simulink model "carsim_seed_model"  (R2024b)
settings: Solver=ode45  StartTime=0  StopTime=12  FixedStep=0.002  RelTol=1e-3  AbsTol=1e-6
libraries: Solver_SF x1
settings Model: Creator=ywata  LastModifiedBy=MrZang
settings SolverCC: AutoScaleAbsTol=off  AlgebraicLoopSolver=TrustRegion
settings DataIOCC: SaveFormat=Array  SignalLoggingSaveFormat=ModelDataLogs  ReturnWorkspaceOutputs=off  SignalLoggingName=sigsOut
settings OptimizationCC: BlockReduction=off  BooleanDataType=off  ExpressionDepthLimit=2147483647  LifeSpan=inf
settings DebuggingCC: SaveWithParameterizedLinksMsg=none  UnderspecifiedInitializationDetection=Classic  MergeDetectMultiDrivingBlocksExec=none  SignalResolutionControl=TryResolveAllWithWarning  MultiTaskDSMMsg=warning  MultiTaskCondExecSysMsg=none  FcnCallInpInsideContextMsg=warning  UnconnectedInputMsg=warning  UnconnectedOutputMsg=warning  UnconnectedLineMsg=warning  StateNameClashWarn=warning  SFUnexpectedBacktrackingDiag=warning  SFNoUnconditionalDefaultTransitionDiag=warning  SFExecutionAtInitializationDiag=none  ArithmeticOperatorsInVariantConditions=warning
settings HardwareCC: ProdBitPerPointer=32  ProdBitPerSizeT=32  ProdBitPerPtrDiffT=32  ProdLargestAtomicFloat=None  ProdIntDivRoundTo=Undefined  ProdEndianess=Unspecified  ProdWordSize=32  ProdHWDeviceType=32-bit Generic  TargetUnknown=on
settings ModelReferenceCC: PropagateSignalLabelsOutOfModel=off
settings SFSimCC: SimUseLocalCustomCode=off  CustomCodeUndefinedFunction=UseInterfaceOnly
settings RTWCC: TemplateMakefile=grt_vc.tmf  RTWUseLocalCustomCode=off  GPUComputeCapability=3.5
settings CodeAppCC: StateflowObjectComments=on
settings GRTTargetCC: TargetFcnLib=ansi_tfl_tmw.mat  TargetLangStandard=C89/C90 (ANSI)  CombineOutputUpdateFcns=off  GRTInterface=on
settings ConfigComp: CovMetricSettings=dw  CovSaveCumulativeToWorkspaceVar=on  CovSaveSingleToWorkspaceVar=on  CovExternalEMLEnable=off

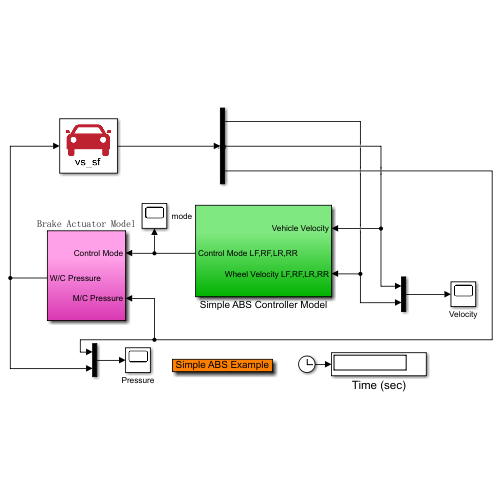
[thumbnail: Simulink's stored preview of the top-level diagram]
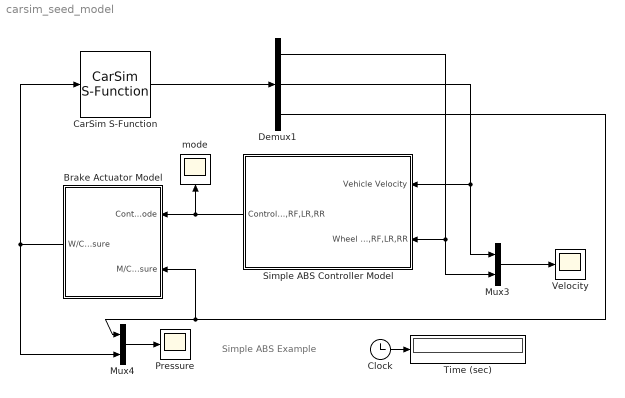
== system carsim_seed_model ==
  note: Simple ABS Example
  Brake Actuator Model : Subsystem
  CarSim S-Function : Solver_SF/CarSim S-Function  Priority=1  SIMFILE=simfile.sim
  Clock : Clock
  Demux1 : Demux  Outputs=[4 1 1]
      settings: DisplayOption=none
  Mux3 : Mux  Inputs=2
  Mux4 : Mux  Inputs=2
  Pressure : Scope
  Simple ABS Controller Model : Subsystem
  Time (sec) : Display
      settings: Format=bank  Decimation=100
  Velocity : Scope
  mode : Scope
  wires:
  Mux4/1 -> Pressure/1
  CarSim S-Function/1 -> Demux1/1
  Demux1/2 -> Mux3/1, Simple ABS Controller Model/1(Vehicle Velocity)
  Demux1/1 -> Mux3/2, Simple ABS Controller Model/2(Wheel Velocity LF,RF,LR,RR)
  Clock/1 -> Time (sec)/1
  Simple ABS Controller Model/1(Control Mode LF,RF,LR,RR) -> Brake Actuator Model/1(Control Mode), mode/1
  Brake Actuator Model/1(W/C Pressure) -> Mux4/2, CarSim S-Function/1
  Mux3/1 -> Velocity/1
  Demux1/3 -> Mux4/1, Brake Actuator Model/2(M/C Pressure)

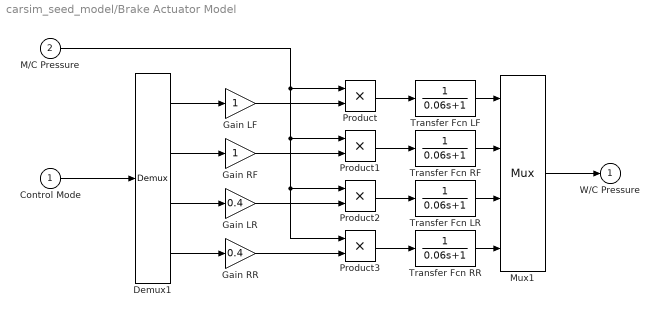
== system carsim_seed_model/Brake Actuator Model ==
  Control Mode : Inport
  M/C Pressure : Inport  Port=2
  Demux1 : Demux
      settings: DisplayOption=none
  Gain LF : Gain  SaturateOnIntegerOverflow=on  OutDataTypeStr=Inherit: Same as input  ParamDataTypeStr=Inherit: Same as input
  Gain LR : Gain  Gain=0.4  SaturateOnIntegerOverflow=on  OutDataTypeStr=Inherit: Same as input  ParamDataTypeStr=Inherit: Same as input
  Gain RF : Gain  SaturateOnIntegerOverflow=on  OutDataTypeStr=Inherit: Same as input  ParamDataTypeStr=Inherit: Same as input
  Gain RR : Gain  Gain=0.4  SaturateOnIntegerOverflow=on  OutDataTypeStr=Inherit: Same as input  ParamDataTypeStr=Inherit: Same as input
  Mux1 : Mux
  Product{,1..3} (4 alike) : Product  InputSameDT=on  SaturateOnIntegerOverflow=on  OutDataTypeStr=Inherit: Same as first input
  Transfer Fcn LF : TransferFcn  Denominator=[0.06 1]
  Transfer Fcn LR : TransferFcn  Denominator=[0.06 1]
  Transfer Fcn RF : TransferFcn  Denominator=[0.06 1]
  Transfer Fcn RR : TransferFcn  Denominator=[0.06 1]
  W/C Pressure : Outport  InitialOutput=0
  wires:
  Mux1/1 -> W/C Pressure/1
  Control Mode/1 -> Demux1/1
  Gain LF/1 -> Product/2
  Gain RF/1 -> Product1/2
  Gain LR/1 -> Product2/2
  Gain RR/1 -> Product3/2
  M/C Pressure/1 -> Product/1, Product1/1, Product2/1, Product3/1
  Product/1 -> Transfer Fcn LF/1
  Transfer Fcn LF/1 -> Mux1/1
  Product1/1 -> Transfer Fcn RF/1
  Product2/1 -> Transfer Fcn LR/1
  Product3/1 -> Transfer Fcn RR/1
  Transfer Fcn RF/1 -> Mux1/2
  Transfer Fcn LR/1 -> Mux1/3
  Transfer Fcn RR/1 -> Mux1/4
  Demux1/1 -> Gain LF/1
  Demux1/2 -> Gain RF/1
  Demux1/3 -> Gain LR/1
  Demux1/4 -> Gain RR/1

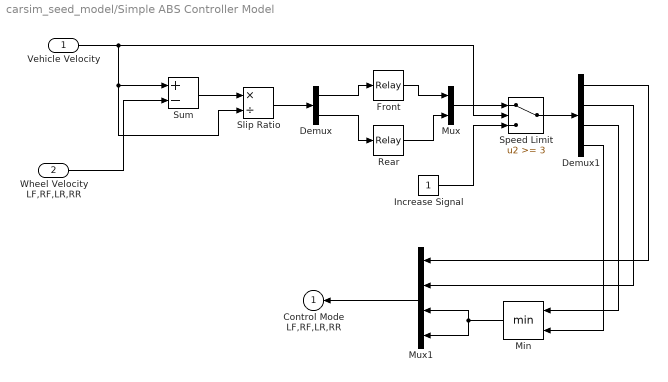
== system carsim_seed_model/Simple ABS Controller Model ==
  Vehicle Velocity : Inport
  Wheel Velocity LF,RF,LR,RR : Inport  Port=2
  Demux : Demux  Outputs=[2 2]
      settings: DisplayOption=none
  Demux1 : Demux
      settings: DisplayOption=none
  Front : Relay  OnSwitchValue=0.1  OffSwitchValue=0.05  OnOutputValue=0  OffOutputValue=1
  Increase Signal : Constant
  Min : MinMax  Inputs=2  InputSameDT=on  SaturateOnIntegerOverflow=on
  Mux : Mux  Inputs=2
  Mux1 : Mux
  Rear : Relay  OnSwitchValue=0.1  OffSwitchValue=0.05  OnOutputValue=0  OffOutputValue=1
  Slip Ratio : Product  Inputs=*/  InputSameDT=on  SaturateOnIntegerOverflow=on  OutDataTypeStr=Inherit: Same as first input
  Speed Limit : Switch  Threshold=3
  Sum : Sum  Inputs=+-  InputSameDT=on  SaturateOnIntegerOverflow=on  OutDataTypeStr=Inherit: Same as first input
  Control Mode LF,RF,LR,RR : Outport  InitialOutput=0
  wires:
  Vehicle Velocity/1 -> Sum/1, Slip Ratio/2, Speed Limit/2
  Speed Limit/1 -> Demux1/1
  Increase Signal/1 -> Speed Limit/3
  Sum/1 -> Slip Ratio/1
  Slip Ratio/1 -> Demux/1
  Mux/1 -> Speed Limit/1
  Min/1 -> Mux1/3, Mux1/4
  Demux1/3 -> Min/1
  Demux1/4 -> Min/2
  Demux1/2 -> Mux1/2
  Demux1/1 -> Mux1/1
  Mux1/1 -> Control Mode LF,RF,LR,RR/1
  Front/1 -> Mux/1
  Demux/1 -> Front/1
  Demux/2 -> Rear/1
  Rear/1 -> Mux/2
  Wheel Velocity LF,RF,LR,RR/1 -> Sum/2
